simulink model "scd3busMicrogridDroopControlFidelityLevels"  (R2025b)
settings: Solver=ode15s  StartTime=0.0  StopTime=48  RelTol=1e-3
PreLoadFcn:
  | scd3busMicrogridDroopControlDataFidelityLevels;
  | 
  | %% Controller variants
  | % Create variant controls for converter controller. Controller has two
  | % different levels of fidelity: Averaged, AveragedPulse, Pulse
  | Averaged = Simulink.VariantExpression;
  | Averaged.Condition = 'fidelity==scd3busMicrogridDroopControl_variants_enum.Low';
  | Pulse = Simulink.VariantExpression;
  | Pulse.Condition = 'fidelity==scd3busMicrogridDroopControl_variants_enum.High';
  | 
  | %% Plant variants
  | % Create variant controls for converter plant. Plant has three different
  | % levels of fidelity.
  | AveragedNonSwitch = Simulink.VariantExpression;
  | AveragedNonSwitch.Condition = 'fidelity==scd3busMicrogridDroopControl_variants_enum.Low';
  | PulseSwitch = Simulink.VariantExpression;
  | PulseSwitch.Condition = 'fidelity==scd3busMicrogridDroopControl_variants_enum.High';
  | 
  | %% Set up variables ready for simulation
  | fidelity = scd3busMicrogridDroopControl_variants_enum.High;
  | Ts = 5e-6;
  | Ts_V = 1e-6;
  | Tsc = 1e-4;
  | Tsc_V = 5e-4;
values from neighbouring files (symbols this model uses):
  consensus = 1    [scd3busMicrogridDroopControlDataFidelityLevels.m]
  fgrid = 60    [scd3busMicrogridDroopControlDataFidelityLevels.m]    (also in scd3busMicrogridDroopControlDataFidelityLevels3Inv.m)
  Kdroop_fp = 0.02/2    (= 0.01)    [scd3busMicrogridDroopControlDataFidelityLevels.m]
  Kdroop_vq = 0.02/2    (= 0.01)    [scd3busMicrogridDroopControlDataFidelityLevels.m]
  Ki_vd = 850    [scd3busMicrogridDroopControlDataFidelityLevels.m]    (also in scd3busMicrogridDroopControlDataFidelityLevels3Inv.m)
  Ki_vq = 850    [scd3busMicrogridDroopControlDataFidelityLevels.m]    (also in scd3busMicrogridDroopControlDataFidelityLevels3Inv.m)
  Kp_vd = 0.36    [scd3busMicrogridDroopControlDataFidelityLevels.m]    (also in scd3busMicrogridDroopControlDataFidelityLevels3Inv.m)
  Kp_vq = 0.36    [scd3busMicrogridDroopControlDataFidelityLevels.m]    (also in scd3busMicrogridDroopControlDataFidelityLevels3Inv.m)
  Ts_DC = 0.001    [scd3busMicrogridDroopControlDataFidelityLevels.m]    (also in scd3busMicrogridDroopControlDataFidelityLevels3Inv.m = 0.0001)
  Vdc1 = 1000    [scd3busMicrogridDroopControlDataFidelityLevels.m]    (also in scd3busMicrogridDroopControlDataFidelityLevels3Inv.m)
  Vdc2 = 1000    [scd3busMicrogridDroopControlDataFidelityLevels.m]    (also in scd3busMicrogridDroopControlDataFidelityLevels3Inv.m)
  Vrms = 380    [scd3busMicrogridDroopControlDataFidelityLevels.m]    (also in scd3busMicrogridDroopControlDataFidelityLevels3Inv.m)
libraries: nesl_utility x60, ee_lib x57, fl_lib x32, eeTransforms x8, eeSinusoidalMeasurement x8, slpidlib x8, eePwmGeneratorTwoLevel x4, eePowerMeasurement x4, simulink x4, SignalEditorBlockLib x1
(part 5 of 5)

== system scd3busMicrogridDroopControlFidelityLevels/Inverter 2/Solar Power 4/MPPT Algorithm ==
  I : Inport
  V : Inport  Port=2
  D_init : Constant  Value=0.611
  D_max : Constant  Value=0.711
  D_min : Constant  Value=0.461
  Delta_D : Constant  Value=0.001
  MPPT Algorithm : MATLAB Function  SystemSampleTime=Ts
  Unit Delay : UnitDelay  InitialCondition=0.5  SampleTime=-1
  Vector Concatenate : Concatenate  NumInputs=4
  duty_cycle : Outport
  wires:
  V/1 -> MPPT Algorithm/2(V)
  Vector Concatenate/1 -> MPPT Algorithm/1(Param)
  D_max/1 -> Vector Concatenate/2
  D_init/1 -> Vector Concatenate/1
  D_min/1 -> Vector Concatenate/3
  MPPT Algorithm/1(D) -> Unit Delay/1
  Delta_D/1 -> Vector Concatenate/4
  I/1 -> MPPT Algorithm/3(I)
  Unit Delay/1 -> duty_cycle/1

== system scd3busMicrogridDroopControlFidelityLevels/Inverter 2/Solar Power 4/Sensing Current ==
  Current Sensor : fl_lib/Electrical/Electrical Sensors/Current Sensor
  PS-Simulink/I : nesl_utility/PS-Simulink Converter  PhysicalDomain=network_engine_domain  SubClassName=ps_output  LeftPortType=input  RightPortType=output  PseudoPeriodic=off  Frequencies=[]  VectorFormat=1-D array  Unit=1  AffineConversion=off
  + : PMIOPort  Side=Left
  - : PMIOPort  Port=2  Side=Right
  I : Outport
  wires:
  PS-Simulink/I/1 -> I/1
  connections:
  -/RConn1 -- Current Sensor/RConn2
  Current Sensor/LConn1 -- +/RConn1
  Current Sensor/RConn1 -- PS-Simulink/I/LConn1

== system scd3busMicrogridDroopControlFidelityLevels/Inverter 2/Solar Power 4/sensing voltage ==
  PS-Simulink Converter : nesl_utility/PS-Simulink Converter  PhysicalDomain=network_engine_domain  SubClassName=ps_output  LeftPortType=input  RightPortType=output  PseudoPeriodic=off  Frequencies=[]  VectorFormat=1-D array  Unit=inherit  AffineConversion=off
  Voltage Sensor : fl_lib/Electrical/Electrical Sensors/Voltage Sensor
  + : PMIOPort  Side=Left
  - : PMIOPort  Port=2  Side=Right
  V : Outport
  wires:
  PS-Simulink Converter/1 -> V/1
  connections:
  Voltage Sensor/LConn1 -- +/RConn1
  Voltage Sensor/RConn2 -- -/RConn1
  Voltage Sensor/RConn1 -- PS-Simulink Converter/LConn1

== system scd3busMicrogridDroopControlFidelityLevels/Inverter 2/Solar Power 4/sensing voltage1 ==
  PS-Simulink Converter : nesl_utility/PS-Simulink Converter  PhysicalDomain=network_engine_domain  SubClassName=ps_output  LeftPortType=input  RightPortType=output  PseudoPeriodic=off  Frequencies=[]  VectorFormat=1-D array  Unit=inherit  AffineConversion=off
  Voltage Sensor : fl_lib/Electrical/Electrical Sensors/Voltage Sensor
  + : PMIOPort  Side=Left
  - : PMIOPort  Port=2  Side=Right
  V : Outport
  wires:
  PS-Simulink Converter/1 -> V/1
  connections:
  Voltage Sensor/LConn1 -- +/RConn1
  Voltage Sensor/RConn2 -- -/RConn1
  Voltage Sensor/RConn1 -- PS-Simulink Converter/LConn1

== system scd3busMicrogridDroopControlFidelityLevels/Inverter 3/Droop Controller Inverter3/DQ Voltage Reference ==
  freq_cmd : Inport
  V_cmd : Inport  Port=2
  Gain : Gain  Gain=2*pi
  Integrator : Integrator
  Product : Product
  Product1 : Product
  Trigonometric Function : Trigonometry
  Trigonometric Function1 : Trigonometry  Operator=cos
  Vd_ref : Outport
  Vq_ref : Outport  Port=2
  wires:
  Product/1 -> Vq_ref/1  "Vq_ref"
  Product1/1 -> Vd_ref/1  "Vd_ref"
  Trigonometric Function/1 -> Product/1
  V_cmd/1 -> Product/2, Product1/1
  Integrator/1 -> Trigonometric Function/1, Trigonometric Function1/1
  freq_cmd/1 -> Gain/1
  Trigonometric Function1/1 -> Product1/2
  Gain/1 -> Integrator/1

== system scd3busMicrogridDroopControlFidelityLevels/Inverter 3/Inverter 3/Averaged Inverter ==
  Averaged Inverter : ee_lib/Semiconductors & Converters/Converters/Converter (Three-Phase)  port_option=ee.enum.threePhasePort.expanded  fidelity_option=ee.enum.converters.fidelity.detailed  device_type=ee.enum.converters.switchingdevice.averaged  showThermalPort=false  K=0  Vth=0.5 V  Vgt=1e-3 V  Vgt_off=-1 V  Ih=1 A  Vf=0.8 V  Ron=1.0000e-03 Ohm  Rds=0.001 Ohm  Goff=2.0000e-04 1/Ohm  Eon_scalar=22.86e-3 J  Eoff_scalar=17.14e-3 J  Eoff_natural_commutation=10e-3 J  Voff=300 V  Iout_scalar=600 A  onCurrentMeasDelay=0 s  useCurrentFromPreviousCycle=false  useVoltageFromPreviousCycle=false  diode_param=ee.enum.converters.protectiondiode.nodynamics  diode_Vf=0.8 V  diode_Ron=0.001 Ohm  diode_Goff=1e-5 1/Ohm  diode_C=50 nF  diode_iRM=-235 A  diode_iF=300 A  diode_idot=-50 A/us  diode_trr_param=ee.enum.converters.diodetrr.trr_factor  diode_trr_factor=3  diode_trr=15 us  diode_Qrr=1.5e+3 s*uA  diode_rec_loss_model=ee.enum.diode.reverseRecoveryModel.fixed  diode_ErecVal=0 J  diode_scaleWithIandV=false  diode_ErecMat=zeros(2, 3) J  diode_TjrecVec=[298.15, 398.15] K  diode_IfrecVec=[.1, 1, 10] A  diode_IrecVal=10 A  diode_VrecVal=10 V  diode_tFilter=1 / 1000 / 100 s  thermal_network_parameterization=ee.enum.thermalNetworkTopology.external  Rth=[.08, .5] K/W  Rth_Cauer=[.08, .1, .5] K/W  Rth_Foster=[.08, .14, .22, .16] K/W  thermal_mass_parameterization=ee.enum.thermalNetwork.timeconstant  thermal_mass=[.01, .5] J/K  thermal_mass_Cauer=[.01, .1, .5] J/K  thermal_mass_Foster=[.001, .005, .05, .5] J/K  thermal_time_constant=[.001, .2] s  thermal_time_constant_Cauer=[.001, .1, .2] s  thermal_time_constant_Foster=[7e-05, .0007, .01, .08] s  thermal_mass_initial_temperatures=[25, 25] degC  thermal_mass_initial_temperatures_Cauer=[25, 25, 25] degC  junction_thermal_mass=0.01 J/K  Tvec_initial_Foster=[25, 25, 25, 25] degC  snubber_type=ee.enum.converters.snubber.exclude  Cs=1e-7 F  Rs=0.1 Ohm  Vce_loss=[0, 150, 300] V
      settings: InternalSimscapePortConfiguration="{\"Bottom\":[],\"Left\":[{\"id\":\"G\",\"label\":\"G\",\"type\":\"foundation.electrical.twelve_phase\"},{\"id\":\"a\",\"label\":\"a\",\"type\":\"foundation.electrical.electrical\"},{\"id\":\"b\",\"label\":\"b\",\"type\":\"foundation.electrical.electrical\"},{\"id\":\"c\",\"label\":\"c\",\"type\":\"foundation.electrical.electrical\"}],\"Right\":[{\"id\":\"p\",\"label\":\"+\",\"type\":\"foundation.electrical.electrical\"},{\"id\":\"n\",\"label\":\"-\",\"type\":\"foundation.electrical.electrical\"}],\"Top\":[]}"
  + : PMIOPort  Side=Right
  G : PMIOPort  Port=2  Side=Left
  a : PMIOPort  Port=3  Side=Left
  b : PMIOPort  Port=4  Side=Left
  - : PMIOPort  Port=5  Side=Right
  c : PMIOPort  Port=6  Side=Left
  connections:
  +/RConn1 -- Averaged Inverter/RConn1
  b/RConn1 -- Averaged Inverter/LConn3
  -/RConn1 -- Averaged Inverter/RConn2
  G/RConn1 -- Averaged Inverter/LConn1
  a/RConn1 -- Averaged Inverter/LConn2
  c/RConn1 -- Averaged Inverter/LConn4

== system scd3busMicrogridDroopControlFidelityLevels/Inverter 3/Inverter 3/IGBT Inverter ==
  IGBT Inverter : ee_lib/Semiconductors & Converters/Converters/Converter (Three-Phase)  port_option=ee.enum.threePhasePort.expanded  fidelity_option=ee.enum.converters.fidelity.detailed  device_type=ee.enum.converters.switchingdevice.igbt  showThermalPort=false  K=0  Vth=0.5 V  Vgt=1e-3 V  Vgt_off=-1 V  Ih=1 A  Vf=0.8 V  Ron=1.0000e-03 Ohm  Rds=0.001 Ohm  Goff=2.0000e-04 1/Ohm  Eon_scalar=22.86e-3 J  Eoff_scalar=17.14e-3 J  Eoff_natural_commutation=10e-3 J  Voff=300 V  Iout_scalar=600 A  onCurrentMeasDelay=0 s  useCurrentFromPreviousCycle=false  useVoltageFromPreviousCycle=false  diode_param=ee.enum.converters.protectiondiode.nodynamics  diode_Vf=0.8 V  diode_Ron=0.001 Ohm  diode_Goff=1e-5 1/Ohm  diode_C=50 nF  diode_iRM=-235 A  diode_iF=300 A  diode_idot=-50 A/us  diode_trr_param=ee.enum.converters.diodetrr.trr_factor  diode_trr_factor=3  diode_trr=15 us  diode_Qrr=1.5e+3 s*uA  diode_rec_loss_model=ee.enum.diode.reverseRecoveryModel.fixed  diode_ErecVal=0 J  diode_scaleWithIandV=false  diode_ErecMat=zeros(2, 3) J  diode_TjrecVec=[298.15, 398.15] K  diode_IfrecVec=[.1, 1, 10] A  diode_IrecVal=10 A  diode_VrecVal=10 V  diode_tFilter=1 / 1000 / 100 s  thermal_network_parameterization=ee.enum.thermalNetworkTopology.external  Rth=[.08, .5] K/W  Rth_Cauer=[.08, .1, .5] K/W  Rth_Foster=[.08, .14, .22, .16] K/W  thermal_mass_parameterization=ee.enum.thermalNetwork.timeconstant  thermal_mass=[.01, .5] J/K  thermal_mass_Cauer=[.01, .1, .5] J/K  thermal_mass_Foster=[.001, .005, .05, .5] J/K  thermal_time_constant=[.001, .2] s  thermal_time_constant_Cauer=[.001, .1, .2] s  thermal_time_constant_Foster=[7e-05, .0007, .01, .08] s  thermal_mass_initial_temperatures=[25, 25] degC  thermal_mass_initial_temperatures_Cauer=[25, 25, 25] degC  junction_thermal_mass=0.01 J/K  Tvec_initial_Foster=[25, 25, 25, 25] degC  snubber_type=ee.enum.converters.snubber.exclude  Cs=1e-7 F  Rs=0.1 Ohm  Vce_loss=[0, 150, 300] V
      settings: InternalSimscapePortConfiguration="{\"Bottom\":[],\"Left\":[{\"id\":\"G\",\"label\":\"G\",\"type\":\"foundation.electrical.twelve_phase\"},{\"id\":\"a\",\"label\":\"a\",\"type\":\"foundation.electrical.electrical\"},{\"id\":\"b\",\"label\":\"b\",\"type\":\"foundation.electrical.electrical\"},{\"id\":\"c\",\"label\":\"c\",\"type\":\"foundation.electrical.electrical\"}],\"Right\":[{\"id\":\"p\",\"label\":\"+\",\"type\":\"foundation.electrical.electrical\"},{\"id\":\"n\",\"label\":\"-\",\"type\":\"foundation.electrical.electrical\"}],\"Top\":[]}"
  + : PMIOPort  Side=Right
  G : PMIOPort  Port=2  Side=Left
  a : PMIOPort  Port=3  Side=Left
  b : PMIOPort  Port=4  Side=Left
  - : PMIOPort  Port=5  Side=Right
  c : PMIOPort  Port=6  Side=Left
  connections:
  c/RConn1 -- IGBT Inverter/LConn4
  a/RConn1 -- IGBT Inverter/LConn2
  G/RConn1 -- IGBT Inverter/LConn1
  -/RConn1 -- IGBT Inverter/RConn2
  b/RConn1 -- IGBT Inverter/LConn3
  +/RConn1 -- IGBT Inverter/RConn1

== system scd3busMicrogridDroopControlFidelityLevels/Inverter 3/Solar Power 3/MPPT Algorithm ==
  I : Inport
  V : Inport  Port=2
  D_init : Constant  Value=0.611
  D_max : Constant  Value=0.711
  D_min : Constant  Value=0.461
  Delta_D : Constant  Value=0.001
  MPPT Algorithm : MATLAB Function  SystemSampleTime=Ts
  Unit Delay : UnitDelay  InitialCondition=0.5  SampleTime=-1
  Vector Concatenate : Concatenate  NumInputs=4
  duty_cycle : Outport
  wires:
  V/1 -> MPPT Algorithm/2(V)
  Vector Concatenate/1 -> MPPT Algorithm/1(Param)
  D_max/1 -> Vector Concatenate/2
  D_init/1 -> Vector Concatenate/1
  D_min/1 -> Vector Concatenate/3
  MPPT Algorithm/1(D) -> Unit Delay/1
  Delta_D/1 -> Vector Concatenate/4
  I/1 -> MPPT Algorithm/3(I)
  Unit Delay/1 -> duty_cycle/1

== system scd3busMicrogridDroopControlFidelityLevels/Inverter 3/Solar Power 3/Sensing Current ==
  Current Sensor : fl_lib/Electrical/Electrical Sensors/Current Sensor
  PS-Simulink/I : nesl_utility/PS-Simulink Converter  PhysicalDomain=network_engine_domain  SubClassName=ps_output  LeftPortType=input  RightPortType=output  PseudoPeriodic=off  Frequencies=[]  VectorFormat=1-D array  Unit=1  AffineConversion=off
  + : PMIOPort  Side=Left
  - : PMIOPort  Port=2  Side=Right
  I : Outport
  wires:
  PS-Simulink/I/1 -> I/1
  connections:
  -/RConn1 -- Current Sensor/RConn2
  Current Sensor/LConn1 -- +/RConn1
  Current Sensor/RConn1 -- PS-Simulink/I/LConn1

== system scd3busMicrogridDroopControlFidelityLevels/Inverter 3/Solar Power 3/sensing voltage ==
  PS-Simulink Converter : nesl_utility/PS-Simulink Converter  PhysicalDomain=network_engine_domain  SubClassName=ps_output  LeftPortType=input  RightPortType=output  PseudoPeriodic=off  Frequencies=[]  VectorFormat=1-D array  Unit=inherit  AffineConversion=off
  Voltage Sensor : fl_lib/Electrical/Electrical Sensors/Voltage Sensor
  + : PMIOPort  Side=Left
  - : PMIOPort  Port=2  Side=Right
  V : Outport
  wires:
  PS-Simulink Converter/1 -> V/1
  connections:
  Voltage Sensor/LConn1 -- +/RConn1
  Voltage Sensor/RConn2 -- -/RConn1
  Voltage Sensor/RConn1 -- PS-Simulink Converter/LConn1

== system scd3busMicrogridDroopControlFidelityLevels/Inverter 3/Solar Power 3/sensing voltage1 ==
  PS-Simulink Converter : nesl_utility/PS-Simulink Converter  PhysicalDomain=network_engine_domain  SubClassName=ps_output  LeftPortType=input  RightPortType=output  PseudoPeriodic=off  Frequencies=[]  VectorFormat=1-D array  Unit=inherit  AffineConversion=off
  Voltage Sensor : fl_lib/Electrical/Electrical Sensors/Voltage Sensor
  + : PMIOPort  Side=Left
  - : PMIOPort  Port=2  Side=Right
  V : Outport
  wires:
  PS-Simulink Converter/1 -> V/1
  connections:
  Voltage Sensor/LConn1 -- +/RConn1
  Voltage Sensor/RConn2 -- -/RConn1
  Voltage Sensor/RConn1 -- PS-Simulink Converter/LConn1

== system scd3busMicrogridDroopControlFidelityLevels/Inverter 4/Droop Controller Inverter3/DQ Voltage Reference ==
  freq_cmd : Inport
  V_cmd : Inport  Port=2
  Gain : Gain  Gain=2*pi
  Integrator : Integrator
  Product : Product
  Product1 : Product
  Trigonometric Function : Trigonometry
  Trigonometric Function1 : Trigonometry  Operator=cos
  Vd_ref : Outport
  Vq_ref : Outport  Port=2
  wires:
  Product/1 -> Vq_ref/1  "Vq_ref"
  Product1/1 -> Vd_ref/1  "Vd_ref"
  Trigonometric Function/1 -> Product/1
  V_cmd/1 -> Product/2, Product1/1
  Integrator/1 -> Trigonometric Function/1, Trigonometric Function1/1
  freq_cmd/1 -> Gain/1
  Trigonometric Function1/1 -> Product1/2
  Gain/1 -> Integrator/1

== system scd3busMicrogridDroopControlFidelityLevels/Inverter 4/Inverter 3/Averaged Inverter ==
  Averaged Inverter : ee_lib/Semiconductors & Converters/Converters/Converter (Three-Phase)  port_option=ee.enum.threePhasePort.expanded  fidelity_option=ee.enum.converters.fidelity.detailed  device_type=ee.enum.converters.switchingdevice.averaged  showThermalPort=false  K=0  Vth=0.5 V  Vgt=1e-3 V  Vgt_off=-1 V  Ih=1 A  Vf=0.8 V  Ron=1.0000e-03 Ohm  Rds=0.001 Ohm  Goff=2.0000e-04 1/Ohm  Eon_scalar=22.86e-3 J  Eoff_scalar=17.14e-3 J  Eoff_natural_commutation=10e-3 J  Voff=300 V  Iout_scalar=600 A  onCurrentMeasDelay=0 s  useCurrentFromPreviousCycle=false  useVoltageFromPreviousCycle=false  diode_param=ee.enum.converters.protectiondiode.nodynamics  diode_Vf=0.8 V  diode_Ron=0.001 Ohm  diode_Goff=1e-5 1/Ohm  diode_C=50 nF  diode_iRM=-235 A  diode_iF=300 A  diode_idot=-50 A/us  diode_trr_param=ee.enum.converters.diodetrr.trr_factor  diode_trr_factor=3  diode_trr=15 us  diode_Qrr=1.5e+3 s*uA  diode_rec_loss_model=ee.enum.diode.reverseRecoveryModel.fixed  diode_ErecVal=0 J  diode_scaleWithIandV=false  diode_ErecMat=zeros(2, 3) J  diode_TjrecVec=[298.15, 398.15] K  diode_IfrecVec=[.1, 1, 10] A  diode_IrecVal=10 A  diode_VrecVal=10 V  diode_tFilter=1 / 1000 / 100 s  thermal_network_parameterization=ee.enum.thermalNetworkTopology.external  Rth=[.08, .5] K/W  Rth_Cauer=[.08, .1, .5] K/W  Rth_Foster=[.08, .14, .22, .16] K/W  thermal_mass_parameterization=ee.enum.thermalNetwork.timeconstant  thermal_mass=[.01, .5] J/K  thermal_mass_Cauer=[.01, .1, .5] J/K  thermal_mass_Foster=[.001, .005, .05, .5] J/K  thermal_time_constant=[.001, .2] s  thermal_time_constant_Cauer=[.001, .1, .2] s  thermal_time_constant_Foster=[7e-05, .0007, .01, .08] s  thermal_mass_initial_temperatures=[25, 25] degC  thermal_mass_initial_temperatures_Cauer=[25, 25, 25] degC  junction_thermal_mass=0.01 J/K  Tvec_initial_Foster=[25, 25, 25, 25] degC  snubber_type=ee.enum.converters.snubber.exclude  Cs=1e-7 F  Rs=0.1 Ohm  Vce_loss=[0, 150, 300] V
      settings: InternalSimscapePortConfiguration="{\"Bottom\":[],\"Left\":[{\"id\":\"G\",\"label\":\"G\",\"type\":\"foundation.electrical.twelve_phase\"},{\"id\":\"a\",\"label\":\"a\",\"type\":\"foundation.electrical.electrical\"},{\"id\":\"b\",\"label\":\"b\",\"type\":\"foundation.electrical.electrical\"},{\"id\":\"c\",\"label\":\"c\",\"type\":\"foundation.electrical.electrical\"}],\"Right\":[{\"id\":\"p\",\"label\":\"+\",\"type\":\"foundation.electrical.electrical\"},{\"id\":\"n\",\"label\":\"-\",\"type\":\"foundation.electrical.electrical\"}],\"Top\":[]}"
  + : PMIOPort  Side=Right
  G : PMIOPort  Port=2  Side=Left
  a : PMIOPort  Port=3  Side=Left
  b : PMIOPort  Port=4  Side=Left
  - : PMIOPort  Port=5  Side=Right
  c : PMIOPort  Port=6  Side=Left
  connections:
  +/RConn1 -- Averaged Inverter/RConn1
  b/RConn1 -- Averaged Inverter/LConn3
  -/RConn1 -- Averaged Inverter/RConn2
  G/RConn1 -- Averaged Inverter/LConn1
  a/RConn1 -- Averaged Inverter/LConn2
  c/RConn1 -- Averaged Inverter/LConn4

== system scd3busMicrogridDroopControlFidelityLevels/Inverter 4/Inverter 3/IGBT Inverter ==
  IGBT Inverter : ee_lib/Semiconductors & Converters/Converters/Converter (Three-Phase)  port_option=ee.enum.threePhasePort.expanded  fidelity_option=ee.enum.converters.fidelity.detailed  device_type=ee.enum.converters.switchingdevice.igbt  showThermalPort=false  K=0  Vth=0.5 V  Vgt=1e-3 V  Vgt_off=-1 V  Ih=1 A  Vf=0.8 V  Ron=1.0000e-03 Ohm  Rds=0.001 Ohm  Goff=2.0000e-04 1/Ohm  Eon_scalar=22.86e-3 J  Eoff_scalar=17.14e-3 J  Eoff_natural_commutation=10e-3 J  Voff=300 V  Iout_scalar=600 A  onCurrentMeasDelay=0 s  useCurrentFromPreviousCycle=false  useVoltageFromPreviousCycle=false  diode_param=ee.enum.converters.protectiondiode.nodynamics  diode_Vf=0.8 V  diode_Ron=0.001 Ohm  diode_Goff=1e-5 1/Ohm  diode_C=50 nF  diode_iRM=-235 A  diode_iF=300 A  diode_idot=-50 A/us  diode_trr_param=ee.enum.converters.diodetrr.trr_factor  diode_trr_factor=3  diode_trr=15 us  diode_Qrr=1.5e+3 s*uA  diode_rec_loss_model=ee.enum.diode.reverseRecoveryModel.fixed  diode_ErecVal=0 J  diode_scaleWithIandV=false  diode_ErecMat=zeros(2, 3) J  diode_TjrecVec=[298.15, 398.15] K  diode_IfrecVec=[.1, 1, 10] A  diode_IrecVal=10 A  diode_VrecVal=10 V  diode_tFilter=1 / 1000 / 100 s  thermal_network_parameterization=ee.enum.thermalNetworkTopology.external  Rth=[.08, .5] K/W  Rth_Cauer=[.08, .1, .5] K/W  Rth_Foster=[.08, .14, .22, .16] K/W  thermal_mass_parameterization=ee.enum.thermalNetwork.timeconstant  thermal_mass=[.01, .5] J/K  thermal_mass_Cauer=[.01, .1, .5] J/K  thermal_mass_Foster=[.001, .005, .05, .5] J/K  thermal_time_constant=[.001, .2] s  thermal_time_constant_Cauer=[.001, .1, .2] s  thermal_time_constant_Foster=[7e-05, .0007, .01, .08] s  thermal_mass_initial_temperatures=[25, 25] degC  thermal_mass_initial_temperatures_Cauer=[25, 25, 25] degC  junction_thermal_mass=0.01 J/K  Tvec_initial_Foster=[25, 25, 25, 25] degC  snubber_type=ee.enum.converters.snubber.exclude  Cs=1e-7 F  Rs=0.1 Ohm  Vce_loss=[0, 150, 300] V
      settings: InternalSimscapePortConfiguration="{\"Bottom\":[],\"Left\":[{\"id\":\"G\",\"label\":\"G\",\"type\":\"foundation.electrical.twelve_phase\"},{\"id\":\"a\",\"label\":\"a\",\"type\":\"foundation.electrical.electrical\"},{\"id\":\"b\",\"label\":\"b\",\"type\":\"foundation.electrical.electrical\"},{\"id\":\"c\",\"label\":\"c\",\"type\":\"foundation.electrical.electrical\"}],\"Right\":[{\"id\":\"p\",\"label\":\"+\",\"type\":\"foundation.electrical.electrical\"},{\"id\":\"n\",\"label\":\"-\",\"type\":\"foundation.electrical.electrical\"}],\"Top\":[]}"
  + : PMIOPort  Side=Right
  G : PMIOPort  Port=2  Side=Left
  a : PMIOPort  Port=3  Side=Left
  b : PMIOPort  Port=4  Side=Left
  - : PMIOPort  Port=5  Side=Right
  c : PMIOPort  Port=6  Side=Left
  connections:
  c/RConn1 -- IGBT Inverter/LConn4
  a/RConn1 -- IGBT Inverter/LConn2
  G/RConn1 -- IGBT Inverter/LConn1
  -/RConn1 -- IGBT Inverter/RConn2
  b/RConn1 -- IGBT Inverter/LConn3
  +/RConn1 -- IGBT Inverter/RConn1

== system scd3busMicrogridDroopControlFidelityLevels/Inverter 4/Solar Power 3/MPPT Algorithm ==
  I : Inport
  V : Inport  Port=2
  D_init : Constant  Value=0.611
  D_max : Constant  Value=0.711
  D_min : Constant  Value=0.461
  Delta_D : Constant  Value=0.001
  MPPT Algorithm : MATLAB Function  SystemSampleTime=Ts
  Unit Delay : UnitDelay  InitialCondition=0.5  SampleTime=-1
  Vector Concatenate : Concatenate  NumInputs=4
  duty_cycle : Outport
  wires:
  V/1 -> MPPT Algorithm/2(V)
  Vector Concatenate/1 -> MPPT Algorithm/1(Param)
  D_max/1 -> Vector Concatenate/2
  D_init/1 -> Vector Concatenate/1
  D_min/1 -> Vector Concatenate/3
  MPPT Algorithm/1(D) -> Unit Delay/1
  Delta_D/1 -> Vector Concatenate/4
  I/1 -> MPPT Algorithm/3(I)
  Unit Delay/1 -> duty_cycle/1

== system scd3busMicrogridDroopControlFidelityLevels/Inverter 4/Solar Power 3/Sensing Current ==
  Current Sensor : fl_lib/Electrical/Electrical Sensors/Current Sensor
  PS-Simulink/I : nesl_utility/PS-Simulink Converter  PhysicalDomain=network_engine_domain  SubClassName=ps_output  LeftPortType=input  RightPortType=output  PseudoPeriodic=off  Frequencies=[]  VectorFormat=1-D array  Unit=1  AffineConversion=off
  + : PMIOPort  Side=Left
  - : PMIOPort  Port=2  Side=Right
  I : Outport
  wires:
  PS-Simulink/I/1 -> I/1
  connections:
  -/RConn1 -- Current Sensor/RConn2
  Current Sensor/LConn1 -- +/RConn1
  Current Sensor/RConn1 -- PS-Simulink/I/LConn1

== system scd3busMicrogridDroopControlFidelityLevels/Inverter 4/Solar Power 3/sensing voltage ==
  PS-Simulink Converter : nesl_utility/PS-Simulink Converter  PhysicalDomain=network_engine_domain  SubClassName=ps_output  LeftPortType=input  RightPortType=output  PseudoPeriodic=off  Frequencies=[]  VectorFormat=1-D array  Unit=inherit  AffineConversion=off
  Voltage Sensor : fl_lib/Electrical/Electrical Sensors/Voltage Sensor
  + : PMIOPort  Side=Left
  - : PMIOPort  Port=2  Side=Right
  V : Outport
  wires:
  PS-Simulink Converter/1 -> V/1
  connections:
  Voltage Sensor/LConn1 -- +/RConn1
  Voltage Sensor/RConn2 -- -/RConn1
  Voltage Sensor/RConn1 -- PS-Simulink Converter/LConn1

== system scd3busMicrogridDroopControlFidelityLevels/Inverter 4/Solar Power 3/sensing voltage1 ==
  PS-Simulink Converter : nesl_utility/PS-Simulink Converter  PhysicalDomain=network_engine_domain  SubClassName=ps_output  LeftPortType=input  RightPortType=output  PseudoPeriodic=off  Frequencies=[]  VectorFormat=1-D array  Unit=inherit  AffineConversion=off
  Voltage Sensor : fl_lib/Electrical/Electrical Sensors/Voltage Sensor
  + : PMIOPort  Side=Left
  - : PMIOPort  Port=2  Side=Right
  V : Outport
  wires:
  PS-Simulink Converter/1 -> V/1
  connections:
  Voltage Sensor/LConn1 -- +/RConn1
  Voltage Sensor/RConn2 -- -/RConn1
  Voltage Sensor/RConn1 -- PS-Simulink Converter/LConn1

== matlab function scd3busMicrogridDroopControlFidelityLevels/Inverter 2/Solar Power 4/MPPT Algorithm/MPPT Algorithm ==
  settings: updateMethod=DISCRETE  sampleTime=Ts_DC
  data: Param input; V input; I input; D output
function D  = PandO(Param, V, I)

% MPPT controller based on the Perturb & Observe algorithm.

% D output = Duty cycle of the boost converter (value between 0 and 1)
%
% V input = PV array terminal voltage (V)
% I input = PV array current (A)
%
% Param input:
Dinit = Param(1);  %Initial value for D output
Dmax = Param(2);   %Maximum value for D
Dmin = Param(3);   %Minimum value for D
deltaD = Param(4); %Increment value used to increase/decrease the duty cycle D
% ( increasing D = decreasing Vref )
%  

persistent Vold Pold Dold;

if isempty(Vold)
    Vold=0;
    Pold=0;
    Dold=Dinit;
end
P= V*I;
dV= V - Vold;
dP= P - Pold;

if dP ~= 0
    %     if dP>1e-9  & dP<-1e-9 & Enabled ~=0
    if dP < 0
        if dV < 0
            D = Dold - deltaD;
        else
            D = Dold + deltaD;
        end
    else
        if dV < 0
            D = Dold + deltaD;
        else
            D = Dold - deltaD;
        end
    end
else
    D = Dold;
end

if D >= Dmax || D<= Dmin
    D = Dold;
end

Dold = D;
Vold = V;
Pold = P;

== matlab function scd3busMicrogridDroopControlFidelityLevels/Inverter 3/Solar Power 3/MPPT Algorithm/MPPT Algorithm ==
  settings: updateMethod=DISCRETE  sampleTime=Ts_DC
  data: Param input; V input; I input; D output
function D  = PandO(Param, V, I)

% MPPT controller based on the Perturb & Observe algorithm.

% D output = Duty cycle of the boost converter (value between 0 and 1)
%
% V input = PV array terminal voltage (V)
% I input = PV array current (A)
%
% Param input:
Dinit = Param(1);  %Initial value for D output
Dmax = Param(2);   %Maximum value for D
Dmin = Param(3);   %Minimum value for D
deltaD = Param(4); %Increment value used to increase/decrease the duty cycle D
% ( increasing D = decreasing Vref )
%  

persistent Vold Pold Dold;

if isempty(Vold)
    Vold=0;
    Pold=0;
    Dold=Dinit;
end
P= V*I;
dV= V - Vold;
dP= P - Pold;

if dP ~= 0
    %     if dP>1e-9  & dP<-1e-9 & Enabled ~=0
    if dP < 0
        if dV < 0
            D = Dold - deltaD;
        else
            D = Dold + deltaD;
        end
    else
        if dV < 0
            D = Dold + deltaD;
        else
            D = Dold - deltaD;
        end
    end
else
    D = Dold;
end

if D >= Dmax || D<= Dmin
    D = Dold;
end

Dold = D;
Vold = V;
Pold = P;

== matlab function scd3busMicrogridDroopControlFidelityLevels/Inverter 4/Solar Power 3/MPPT Algorithm/MPPT Algorithm ==
  settings: updateMethod=DISCRETE  sampleTime=Ts_DC
  data: Param input; V input; I input; D output
function D  = PandO(Param, V, I)

% MPPT controller based on the Perturb & Observe algorithm.

% D output = Duty cycle of the boost converter (value between 0 and 1)
%
% V input = PV array terminal voltage (V)
% I input = PV array current (A)
%
% Param input:
Dinit = Param(1);  %Initial value for D output
Dmax = Param(2);   %Maximum value for D
Dmin = Param(3);   %Minimum value for D
deltaD = Param(4); %Increment value used to increase/decrease the duty cycle D
% ( increasing D = decreasing Vref )
%  

persistent Vold Pold Dold;

if isempty(Vold)
    Vold=0;
    Pold=0;
    Dold=Dinit;
end
P= V*I;
dV= V - Vold;
dP= P - Pold;

if dP ~= 0
    %     if dP>1e-9  & dP<-1e-9 & Enabled ~=0
    if dP < 0
        if dV < 0
            D = Dold - deltaD;
        else
            D = Dold + deltaD;
        end
    else
        if dV < 0
            D = Dold + deltaD;
        else
            D = Dold - deltaD;
        end
    end
else
    D = Dold;
end

if D >= Dmax || D<= Dmin
    D = Dold;
end

Dold = D;
Vold = V;
Pold = P;

== matlab function scd3busMicrogridDroopControlFidelityLevels/Droop Controller Inverter1/MATLAB Function ==
  settings: updateMethod=DISCRETE  sampleTime=0.5
  data: freq_i input; delta_P0 output; V_i input; freq_inv2 input; freq_inv3 input; freq_inv4 input; V_inv2 input; V_inv3 input; delta_Q0 output; V_inv4 input; xi_f_prev input; xi_V_prev input; consensus_enable input; xi_f_next output; xi_V_next output
%% ----------------------------------------------------------
%  AGENT 1 — INVERTOR 1  (versiune PI consensus)
%  Vecini: Inv2, Inv3, Inv4
%
%  INTRĂRI:
%    freq_i, V_i          — măsurători locale (de la PLL)
%    freq_inv2..4         — frecvențele vecinilor (communication link)
%    V_inv2..4            — tensiunile vecinilor (communication link)
%    xi_f_prev            — starea integratorului de frecvență (Unit Delay)
%    xi_V_prev            — starea integratorului de tensiune (Unit Delay)
%    consensus_enable     — flag 0/1 (din scriptul tău: variabila "consensus")
%
%  IEȘIRI:
%    delta_P0             — corecție setpoint putere activă [pu]
%    delta_Q0             — corecție setpoint putere reactivă [pu]
%    xi_f_next            — starea actualizată a integratorului f (→ Unit Delay)
%    xi_V_next            — starea actualizată a integratorului V (→ Unit Delay)
%% ----------------------------------------------------------

function [delta_P0, delta_Q0, xi_f_next, xi_V_next] = consensus_inv1(...
    freq_i,   V_i,       ...
    freq_inv2, freq_inv3, freq_inv4, ...
    V_inv2,    V_inv3,    V_inv4,    ...
    xi_f_prev, xi_V_prev,            ...
    consensus_enable)

%% ── PARAMETRI ──────────────────────────────────────────────

f_nom   = 60.0;     % Frecvența nominală [Hz]
V_nom   = 1.0;      % Tensiunea nominală [pu]

% Gains consensus frecvență
Kp_f    = 0.02;     % Gain proportional  (sincronizare peer-to-peer)
Ki_f    = 0.05;     % Gain integral      (restaurare la f_nom)

% Gains consensus tensiune
Kp_V    = 0.05;     % Gain proportional
Ki_V    = 0.10;     % Gain integral

% Sample time al blocului MATLAB Function
%   Trebuie să fie ACELAȘI cu Ts_DC din script (0.001 s)
Tsc     = 0.001;

% Limite saturație ieșiri
dP0_lim = 0.20;     % [pu] — max 20% corecție față de P0
dQ0_lim = 0.10;     % [pu] — max 10% corecție față de Q0

% Limite saturație integratoare (anti-windup)
xi_f_lim = 0.15;    % [pu]
xi_V_lim = 0.08;    % [pu]

%% ── TERMENUL DE CONSENS (peer-to-peer) ──────────────────────
% Aceasta e componenta proportionala — sincronizare intre vecini
% Fiecare vecin contribuie egal (weight = 1, graf neponderat)

sum_freq = (freq_inv2 - freq_i) + ...
           (freq_inv3 - freq_i) + ...
           (freq_inv4 - freq_i);

sum_V    = (V_inv2 - V_i) + ...
           (V_inv3 - V_i) + ...
           (V_inv4 - V_i);

%% ── TERMENUL DE TRACKING (eroarea față de nominal) ───────────
% Aceasta e componenta integrala — restaurare la valoarea nominala
% Fara aceasta, consensul pur poate sincroniza invertoarele
% la o frecventa gresita (ex: toti la 59.7Hz in loc de 60Hz)

err_f = f_nom - freq_i;   % pozitiv când freq e sub nominal
err_V = V_nom - V_i;      % pozitiv când tensiunea e sub nominal

%% ── ACTUALIZARE INTEGRATOARE (Euler forward) ────────────────
% Formula: xi[k] = xi[k-1] + Tsc * Ki * eroare[k]
% Anti-windup: saturăm starea integratorului, nu doar ieșirea

xi_f_raw = xi_f_prev + Tsc * Ki_f * err_f;
xi_V_raw = xi_V_prev + Tsc * Ki_V * err_V;

% Saturație integratoare (anti-windup clamping)
xi_f_next = max(min(xi_f_raw, xi_f_lim), -xi_f_lim);
xi_V_next = max(min(xi_V_raw, xi_V_lim), -xi_V_lim);

%% ── IEȘIRI TOTALE ────────────────────────────────────────────
% Componenta P  = proportional (consens) + integral (tracking)
% Structura PI distribuita:
%   delta_P0 = Kp * Σ(freq_j - freq_i)  +  xi_f
%   delta_Q0 = Kp * Σ(V_j - V_i)        +  xi_V

if consensus_enable

    dP0_raw = Kp_f * sum_freq + xi_f_next;
    dQ0_raw = Kp_V * sum_V    + xi_V_next;

    % Saturatie iesire finala
    delta_P0 = max(min(dP0_raw, dP0_lim), -dP0_lim);
    delta_Q0 = max(min(dQ0_raw, dQ0_lim), -dQ0_lim);

else
    % Consensul dezactivat — droop clasic pur
    delta_P0 = 0;
    delta_Q0 = 0;
end

end

== matlab function scd3busMicrogridDroopControlFidelityLevels/Inverter 2/Droop Controller Inverter2/MATLAB Function ==
  settings: updateMethod=DISCRETE  sampleTime=0.5
  data: freq_i input; delta_P0 output; V_i input; freq_inv1 input; freq_inv3 input; freq_inv4 input; V_inv1 input; V_inv3 input; delta_Q0 output; V_inv4 input; xi_f_prev input; xi_V_prev input; consensus_enable input; xi_f_next output; xi_V_next output
%% ----------------------------------------------------------
%  AGENT 2 — INVERTOR 2  (versiune PI consensus)
%  Vecini: Inv1, Inv3, Inv4
%
%  INTRĂRI:
%    freq_i, V_i          — măsurători locale
%    freq_inv1,3,4        — frecvențele vecinilor
%    V_inv1,3,4           — tensiunile vecinilor
%    xi_f_prev            — starea integratorului f (Unit Delay)
%    xi_V_prev            — starea integratorului V (Unit Delay)
%    consensus_enable     — flag 0/1
%% ----------------------------------------------------------

function [delta_P0, delta_Q0, xi_f_next, xi_V_next] = consensus_inv2(...
    freq_i,    V_i,       ...
    freq_inv1, freq_inv3, freq_inv4, ...
    V_inv1,    V_inv3,    V_inv4,    ...
    xi_f_prev, xi_V_prev,            ...
    consensus_enable)

%% ── PARAMETRI ──────────────────────────────────────────────
% IDENTICI cu Inv1 — sistem simetric
f_nom    = 60.0;
V_nom    = 1.0;

Kp_f     = 0.02;
Ki_f     = 0.05;
Kp_V     = 0.05;
Ki_V     = 0.10;

Tsc      = 0.001;

dP0_lim  = 0.20;
dQ0_lim  = 0.10;
xi_f_lim = 0.15;
xi_V_lim = 0.08;

%% ── TERMEN CONSENS peer-to-peer ─────────────────────────────
% Vecini: Inv1, Inv3, Inv4 (diferit față de Inv1 care vedea Inv2,3,4)
sum_freq = (freq_inv1 - freq_i) + ...
           (freq_inv3 - freq_i) + ...
           (freq_inv4 - freq_i);

sum_V    = (V_inv1 - V_i) + ...
           (V_inv3 - V_i) + ...
           (V_inv4 - V_i);

%% ── EROARE FAȚĂ DE NOMINAL ──────────────────────────────────
err_f = f_nom - freq_i;
err_V = V_nom - V_i;

%% ── ACTUALIZARE INTEGRATOARE ────────────────────────────────
xi_f_raw  = xi_f_prev + Tsc * Ki_f * err_f;
xi_V_raw  = xi_V_prev + Tsc * Ki_V * err_V;

xi_f_next = max(min(xi_f_raw,  xi_f_lim), -xi_f_lim);
xi_V_next = max(min(xi_V_raw,  xi_V_lim), -xi_V_lim);

%% ── IEȘIRI ──────────────────────────────────────────────────
if consensus_enable

    dP0_raw  = Kp_f * sum_freq + xi_f_next;
    dQ0_raw  = Kp_V * sum_V    + xi_V_next;

    delta_P0 = max(min(dP0_raw, dP0_lim), -dP0_lim);
    delta_Q0 = max(min(dQ0_raw, dQ0_lim), -dQ0_lim);

else
    delta_P0 = 0;
    delta_Q0 = 0;
end

end

== matlab function scd3busMicrogridDroopControlFidelityLevels/Inverter 3/Droop Controller Inverter3/MATLAB Function ==
  settings: updateMethod=DISCRETE  sampleTime=0.5
  data: freq_i input; delta_P0 output; V_i input; freq_inv1 input; freq_inv2 input; freq_inv4 input; V_inv1 input; V_inv2 input; delta_Q0 output; V_inv4 input; xi_f_prev input; xi_V_prev input; consensus_enable input; xi_f_next output; xi_V_next output
%% ----------------------------------------------------------
%  AGENT 3 — INVERTOR 3  (versiune PI consensus)
%  Vecini: Inv1, Inv2, Inv4
%% ----------------------------------------------------------

function [delta_P0, delta_Q0, xi_f_next, xi_V_next] = consensus_inv3(...
    freq_i,    V_i,       ...
    freq_inv1, freq_inv2, freq_inv4, ...
    V_inv1,    V_inv2,    V_inv4,    ...
    xi_f_prev, xi_V_prev,            ...
    consensus_enable)

%% ── PARAMETRI ──────────────────────────────────────────────
f_nom    = 60.0;
V_nom    = 1.0;

Kp_f     = 0.02;
Ki_f     = 0.05;
Kp_V     = 0.05;
Ki_V     = 0.10;

Tsc      = 0.001;

dP0_lim  = 0.20;
dQ0_lim  = 0.10;
xi_f_lim = 0.15;
xi_V_lim = 0.08;

%% ── TERMEN CONSENS peer-to-peer ─────────────────────────────
sum_freq = (freq_inv1 - freq_i) + ...
           (freq_inv2 - freq_i) + ...
           (freq_inv4 - freq_i);

sum_V    = (V_inv1 - V_i) + ...
           (V_inv2 - V_i) + ...
           (V_inv4 - V_i);

%% ── EROARE FAȚĂ DE NOMINAL ──────────────────────────────────
err_f = f_nom - freq_i;
err_V = V_nom - V_i;

%% ── ACTUALIZARE INTEGRATOARE ────────────────────────────────
xi_f_raw  = xi_f_prev + Tsc * Ki_f * err_f;
xi_V_raw  = xi_V_prev + Tsc * Ki_V * err_V;

xi_f_next = max(min(xi_f_raw,  xi_f_lim), -xi_f_lim);
xi_V_next = max(min(xi_V_raw,  xi_V_lim), -xi_V_lim);

%% ── IEȘIRI ──────────────────────────────────────────────────
if consensus_enable

    dP0_raw  = Kp_f * sum_freq + xi_f_next;
    dQ0_raw  = Kp_V * sum_V    + xi_V_next;

    delta_P0 = max(min(dP0_raw, dP0_lim), -dP0_lim);
    delta_Q0 = max(min(dQ0_raw, dQ0_lim), -dQ0_lim);

else
    delta_P0 = 0;
    delta_Q0 = 0;
end

end

== matlab function scd3busMicrogridDroopControlFidelityLevels/Inverter 4/Droop Controller Inverter3/MATLAB Function ==
  settings: updateMethod=DISCRETE  sampleTime=0.5
  data: freq_i input; delta_P0 output; V_i input; freq_inv1 input; freq_inv2 input; freq_inv3 input; V_inv1 input; V_inv2 input; delta_Q0 output; V_inv3 input; xi_f_prev input; xi_V_prev input; consensus_enable input; xi_f_next output; xi_V_next output
%% ----------------------------------------------------------
%  AGENT 4 — INVERTOR 4  (versiune PI consensus)
%  Vecini: Inv1, Inv2, Inv3
%% ----------------------------------------------------------

function [delta_P0, delta_Q0, xi_f_next, xi_V_next] = consensus_inv4(...
    freq_i,    V_i,       ...
    freq_inv1, freq_inv2, freq_inv3, ...
    V_inv1,    V_inv2,    V_inv3,    ...
    xi_f_prev, xi_V_prev,            ...
    consensus_enable)

%% ── PARAMETRI ──────────────────────────────────────────────
f_nom    = 60.0;
V_nom    = 1.0;

Kp_f     = 0.02;
Ki_f     = 0.05;
Kp_V     = 0.05;
Ki_V     = 0.10;

Tsc      = 0.001;

dP0_lim  = 0.20;
dQ0_lim  = 0.10;
xi_f_lim = 0.15;
xi_V_lim = 0.08;

%% ── TERMEN CONSENS peer-to-peer ─────────────────────────────
sum_freq = (freq_inv1 - freq_i) + ...
           (freq_inv2 - freq_i) + ...
           (freq_inv3 - freq_i);

sum_V    = (V_inv1 - V_i) + ...
           (V_inv2 - V_i) + ...
           (V_inv3 - V_i);

%% ── EROARE FAȚĂ DE NOMINAL ──────────────────────────────────
err_f = f_nom - freq_i;
err_V = V_nom - V_i;

%% ── ACTUALIZARE INTEGRATOARE ────────────────────────────────
xi_f_raw  = xi_f_prev + Tsc * Ki_f * err_f;
xi_V_raw  = xi_V_prev + Tsc * Ki_V * err_V;

xi_f_next = max(min(xi_f_raw,  xi_f_lim), -xi_f_lim);
xi_V_next = max(min(xi_V_raw,  xi_V_lim), -xi_V_lim);

%% ── IEȘIRI ──────────────────────────────────────────────────
if consensus_enable

    dP0_raw  = Kp_f * sum_freq + xi_f_next;
    dQ0_raw  = Kp_V * sum_V    + xi_V_next;

    delta_P0 = max(min(dP0_raw, dP0_lim), -dP0_lim);
    delta_Q0 = max(min(dQ0_raw, dQ0_lim), -dQ0_lim);

else
    delta_P0 = 0;
    delta_Q0 = 0;
end

end

== matlab function scd3busMicrogridDroopControlFidelityLevels/Solar Power 1/MPPT Algorithm/MPPT Algorithm ==
  settings: updateMethod=DISCRETE  sampleTime=Ts_DC
  data: Param input; V input; I input; D output
function D  = PandO(Param, V, I)

% MPPT controller based on the Perturb & Observe algorithm.

% D output = Duty cycle of the boost converter (value between 0 and 1)
%
% V input = PV array terminal voltage (V)
% I input = PV array current (A)
%
% Param input:
Dinit = Param(1);  %Initial value for D output
Dmax = Param(2);   %Maximum value for D
Dmin = Param(3);   %Minimum value for D
deltaD = Param(4); %Increment value used to increase/decrease the duty cycle D
% ( increasing D = decreasing Vref )
%  

persistent Vold Pold Dold;

if isempty(Vold)
    Vold=0;
    Pold=0;
    Dold=Dinit;
end
P= V*I;
dV= V - Vold;
dP= P - Pold;

if dP ~= 0
    %     if dP>1e-9  & dP<-1e-9 & Enabled ~=0
    if dP < 0
        if dV < 0
            D = Dold - deltaD;
        else
            D = Dold + deltaD;
        end
    else
        if dV < 0
            D = Dold + deltaD;
        else
            D = Dold - deltaD;
        end
    end
else
    D = Dold;
end

if D >= Dmax || D<= Dmin
    D = Dold;
end

Dold = D;
Vold = V;
Pold = P;
